simulink model "final"  (R2024b)
settings: Solver=ode23t  StartTime=0.0  StopTime=0.5  RelTol=1e-3
libraries: spsSeriesRLCBranchLib x4, spsRMSLib x2, spsCurrentMeasurementLib x1, spsDiodeLib x1, spsIGBTDiodeLib x1, spsPVArrayLib x1, slpidlib x1, simulink x1, spsVoltageMeasurementLib x1, sps_lib x1
settings Model: Creator=Aamith Kishore T J  LastModifiedBy=Aamith Kishore T J

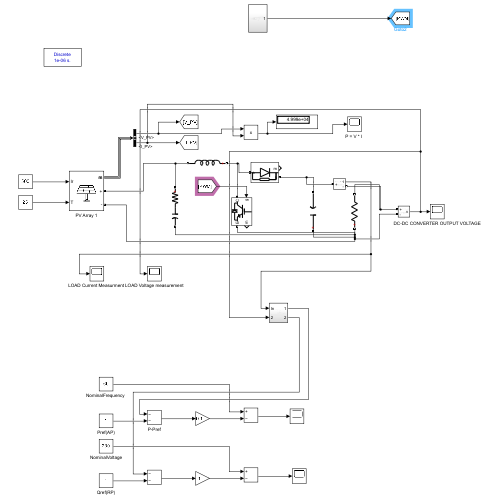
[thumbnail: Simulink's stored preview of the top-level diagram]
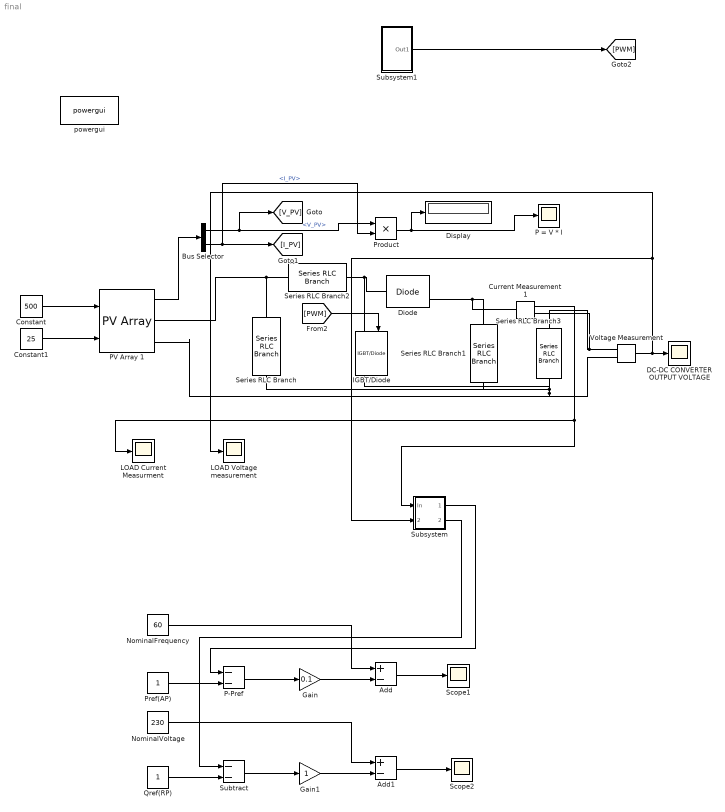
== system final ==
  Add : Sum  Inputs=+-
  Add1 : Sum  Inputs=+-
  Bus Selector : BusSelector  OutputSignals=V_PV,I_PV
  Constant : Constant  Value=500
  Constant1 : Constant  Value=25
  Current Measurement1 : spsCurrentMeasurementLib/Current Measurement  PhasorSimulation=off  OutputType=Complex  PSBequivalent=0
  DC-DC CONVERTER OUTPUT VOLTAGE : Scope
  Diode : spsDiodeLib/Diode  Ron=0.001  Lon=0  Vf=0.8  IC=0  UseSnubber=0  Rs=500  Cs=250e-9  Measurements=on
  Display : Display
  Gain : Gain  Gain=0.1
  Gain1 : Gain
  IGBT/Diode : spsIGBTDiodeLib/IGBT//Diode  Ron=1e-3  Rs=1e5  Cs=inf  Measurements=on
  "LOAD Current Measurment " : Scope
  LOAD Voltage measurement : Scope
  "NominalFrequency " : Constant  Value=60
  NominalVoltage : Constant  Value=230
  "P = V * I " : Scope
  P-Pref : Sum  Inputs=--
  PV Array 1 : spsPVArrayLib/PV Array  Npar=47  Nser=10  PlotType=array @ 25 deg.C & specified irradiances  S_vec="[ 1000  500  100 ]"  Temp_C_vec=[25 0]  ModuleName=A2Peak Power POWER ON P220-6x10  PlotWhenSelected=off  Pm=219.978  Ncell=60  Voc=36.72  Isc=7.98  Vm=30.3  Im=7.26  beta_Voc_pc=-0.35  alpha_Isc_pc=0.05  beta_Voc=-0.12852  alpha_Isc=0.00399  IL=8.0041  I0=1.8441e-10  nI=0.97472  Rsh=85.0716  Rs=0.25728  RobustModel=off  RobustCellTemperature=313.3991  BAL=on  Tc=1e-6  Tfilter=5e-5
  Pref(AP) : Constant
  Product : Product
  Qref(RP) : Constant
  Scope1 : Scope
  Scope2 : Scope
  Series RLC Branch : spsSeriesRLCBranchLib/Series RLC Branch  LConnTagsString=__new0  RConnTagsString=__new0  BranchType=RC  Resistance=0.0001  Inductance=1e-3  SetiL0=off  InitialCurrent=0  Capacitance=1000e-6  Setx0=off  InitialVoltage=0  Measurements=None
  Series RLC Branch1 : spsSeriesRLCBranchLib/Series RLC Branch  LConnTagsString=__new0  RConnTagsString=__new0  BranchType=C  Resistance=0.0001  Inductance=1.45e-6  SetiL0=off  InitialCurrent=0  Capacitance=3227e-6  Setx0=off  InitialVoltage=0  Measurements=None
  Series RLC Branch2 : spsSeriesRLCBranchLib/Series RLC Branch  LConnTagsString=__new0  RConnTagsString=__new0  BranchType=L  Resistance=0.0001  Inductance=1.45e-6  SetiL0=off  InitialCurrent=0  Capacitance=9888-6  Setx0=off  InitialVoltage=0  Measurements=None
  Series RLC Branch3 : spsSeriesRLCBranchLib/Series RLC Branch  LConnTagsString=__new0  RConnTagsString=__new0  BranchType=R  Resistance=2  Inductance=1.45e-6  SetiL0=off  InitialCurrent=0  Capacitance=3227e-6  Setx0=off  InitialVoltage=0  Measurements=None
  Subsystem : Subsystem
  Subsystem1 : Subsystem
  Subtract : Sum  Inputs=--
  Voltage Measurement : spsVoltageMeasurementLib/Voltage Measurement  PhasorSimulation=off  OutputType=Complex  PSBequivalent=0
  powergui : sps_lib/powergui  Priority=1  SimulationMode=Discrete  SampleTime=1e-6  frequency=60  Iterations=50  frequencyindice=0  Pbase=100e6  ErrMax=1e-4  UnitsV=kV  UnitsW=MW  buscounter=0  FunctionMessages=off  echomessages=off  EnableUseOfTLC=off  CurrentSourceSwitches=off  DisableSnubberDevices=off  DisableRonSwitches=off  DisableVfSwitches=off  DisplayEquations=off  AutomaticDiscreteSolvers=off  SolverType=Tustin/Backward Euler (TBE)  Interpol=off  ExternalGateDelay=off  methode=off  Ts=100  x0status=blocks  SPID=on  SwTol=0  HookPort=off  NonlinearTolerance=1e-4  nMaxIteration=100  ContinueOnMaxIteration=off  RestoreLinks=warning  ResistiveCurrentMeasurement=off  Frange=[0:2:500]  Ylog=off  Xlog=on  ShowGrid=off  save=off  variable=ZData  structure=0  ZoomFFT=off  StartTime=0.0  cycles=1  DisplayStyle=1  fundamental=60  FreqAxis=off  MaxFrequency=1000  frequencyindicesteady=1  RmsSteady=1  display=off
  wires:
  Constant/1 -> PV Array 1/1
  Constant1/1 -> PV Array 1/2
  PV Array 1/1 -> Bus Selector/1
  Bus Selector/1 -> Product/1, [V_PV]  "<V_PV>"
  Bus Selector/2 -> Product/2, [I_PV]  "<I_PV>"
  [PWM] -> IGBT/Diode/1
  Product/1 -> "P = V * I "/1, Display/1
  P-Pref/1 -> Gain/1
  Pref(AP)/1 -> P-Pref/2
  "NominalFrequency "/1 -> Add/1
  Gain/1 -> Add/2
  Add/1 -> Scope1/1
  Qref(RP)/1 -> Subtract/2
  Subtract/1 -> Gain1/1
  NominalVoltage/1 -> Add1/1
  Gain1/1 -> Add1/2
  Add1/1 -> Scope2/1
  Voltage Measurement/1 -> Subsystem/2(In1), LOAD Voltage measurement/1, DC-DC CONVERTER OUTPUT VOLTAGE/1
  Current Measurement1/1 -> Subsystem/1(In), "LOAD Current Measurment "/1
  Subsystem/1(Out1) -> P-Pref/1
  Subsystem/2(Out2) -> Subtract/1
  Subsystem1/1(Out1) -> [PWM]
  connections:
  PV Array 1/RConn1 -- Series RLC Branch2/RConn1 -- Series RLC Branch/LConn1
  Series RLC Branch/RConn1 -- Voltage Measurement/LConn2 -- PV Array 1/RConn2 -- Series RLC Branch1/LConn1 -- IGBT/Diode/RConn1 -- Series RLC Branch3/LConn1
  Diode/LConn1 -- Series RLC Branch2/LConn1 -- IGBT/Diode/LConn1
  Diode/RConn1 -- Current Measurement1/LConn1 -- Series RLC Branch1/RConn1
  Series RLC Branch3/RConn1 -- Voltage Measurement/LConn1 -- Current Measurement1/RConn1

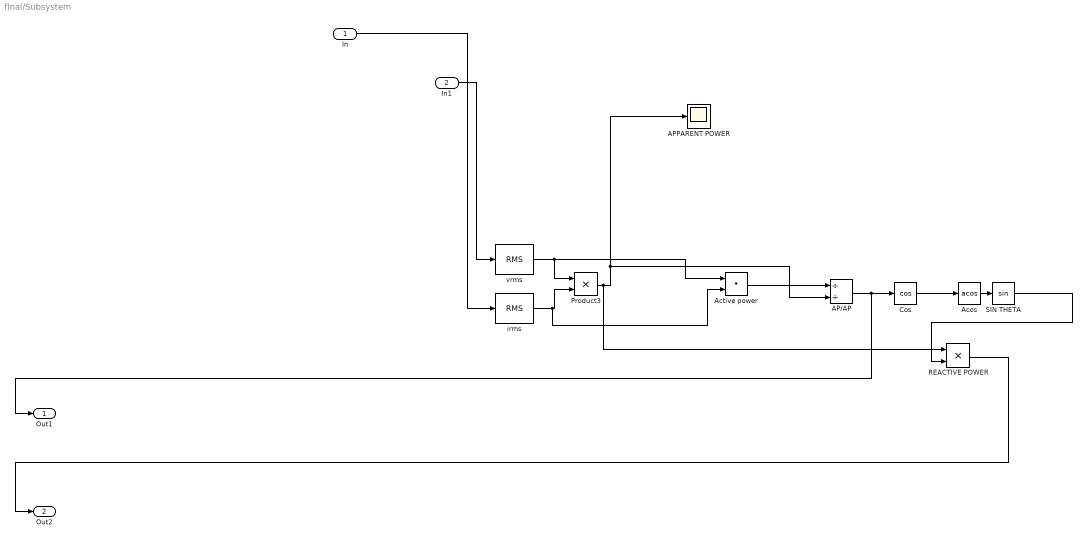
== system final/Subsystem ==
  In : Inport
  In1 : Inport  Port=2
  AP/AP : Product  Inputs=//
  APPARENT POWER : Scope
  Acos : Trigonometry  Operator=acos
  Active power : DotProduct  OutDataTypeStr=Inherit: Inherit via internal rule
  Cos : Trigonometry  Operator=cos
  Product3 : Product
  REACTIVE POWER : Product
  SIN THETA : Trigonometry
  irms : spsRMSLib/RMS  TrueRMS=on  Freq=60  RMSInit=120  Ts=0
  vrms : spsRMSLib/RMS  TrueRMS=on  Freq=60  RMSInit=120  Ts=0
  Out1 : Outport
  Out2 : Outport  Port=2
  wires:
  Acos/1 -> SIN THETA/1
  irms/1 -> Active power/2, Product3/2
  AP/AP/1 -> Out1/1, Cos/1
  vrms/1 -> Active power/1, Product3/1
  SIN THETA/1 -> REACTIVE POWER/2
  Active power/1 -> AP/AP/1
  In1/1 -> vrms/1
  Product3/1 -> REACTIVE POWER/1, AP/AP/2, APPARENT POWER/1
  REACTIVE POWER/1 -> Out2/1
  Cos/1 -> Acos/1
  In/1 -> irms/1

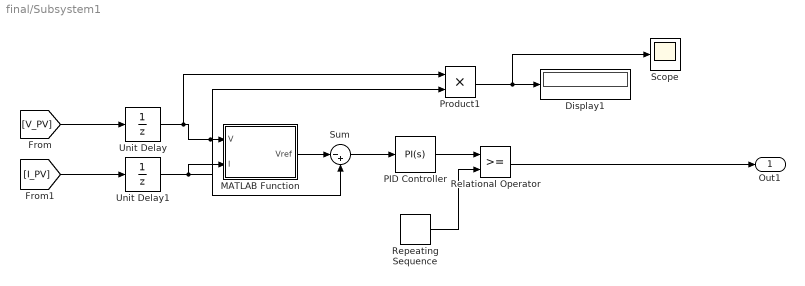
== system final/Subsystem1 ==
  Display1 : Display
  MATLAB Function : MATLAB Function  TreatAsAtomicUnit=on
  PID Controller : slpidlib/PID Controller  Controller=PI  Form=Parallel  TimeDomain=Continuous-time  UseExternalTs=off  SampleTime=-1  IntegratorMethod=Forward Euler  FilterMethod=Forward Euler  ControllerParametersSource=internal  P=0.001  I=0.01  UseKiTs=off  D=0  UseExternalDerivativeSource=off  N=100  UseFilter=on  TunerSelectOption=Transfer Function Based (PID Tuner App)  InitialConditionSource=internal  InitialConditionForIntegrator=0  InitialConditionForFilter=0  DifferentiatorICPrevScaledInput=0  ExternalReset=none  TrackingMode=off  Kt=1  LimitOutput=on  SatLimitsSource=internal  UpperSaturationLimit=0.95  LowerSaturationLimit=0  LinearizeAsGain=on  AntiWindupMode=none  Kb=1  LimitIntegrator=off  UpperIntegratorSaturationLimit=inf  LowerIntegratorSaturationLimit=-inf  POutMin=[]  POutMax=[]  IOutMin=[]  IOutMax=[]  DOutMin=[]  DOutMax=[]  NOutMin=[]  NOutMax=[]  SumOutMin=[]  SumOutMax=[]  SaturationOutMin=[]  SaturationOutMax=[]  PParamMin=[]  PParamMax=[]  IParamMin=[]  IParamMax=[]  DParamMin=[]  DParamMax=[]  NParamMin=[]  NParamMax=[]  KbParamMin=[]  KbParamMax=[]  KtParamMin=[]  KtParamMax=[]  KbOutMin=[]  KbOutMax=[]  KtOutMin=[]  KtOutMax=[]  IntegratorOutMin=[]  IntegratorOutMax=[]  FilterOutMin=[]  FilterOutMax=[]  SumI1OutMin=[]  SumI1OutMax=[]  SumI2OutMin=[]  SumI2OutMax=[]  SumI3OutMin=[]  SumI3OutMax=[]  SumI4OutMin=[]  SumI4OutMax=[]  SumDOutMin=[]  SumDOutMax=[]  DifferentiatorOutMin=[]  DifferentiatorOutMax=[]  FilterDiffOutCoefMin=[]  FilterDiffOutCoefMax=[]  ReciprocalOutMin=[]  ReciprocalOutMax=[]  SumDenOutMin=[]  SumDenOutMax=[]  SumNumOutMin=[]  SumNumOutMax=[]  DivideOutMin=[]  DivideOutMax=[]  UdiffTsProdOutMin=[]  UdiffTsProdOutMax=[]  NTsProdOutMin=[]  NTsProdOutMax=[]  UintegralTsProdOutMin=[]  UintegralTsProdOutMax=[]  UngainTsProdOutMin=[]  UngainTsProdOutMax=[]  ClampingZeroOutDataTypeStr=Inherit: Inherit via back propagation  ClampingZeroOutMin=[]  ClampingZeroOutMax=[]  FilterDenConstantOutDataTypeStr=Inherit: Inherit via back propagation  FilterDenConstantOutMin=[]  FilterDenConstantOutMax=[]  PCopyOutDataTypeStr=Inherit: Inherit via back propagation  PCopyOutMin=[]  PCopyOutMax=[]  NCopyOutDataTypeStr=Inherit: Inherit via back propagation  NCopyOutMin=[]  NCopyOutMax=[]  IntegratorContinuousStateAttributes=''  IntegratorStateMustResolveToSignalObject=off  IntegratorRTWStateStorageClass=Auto  FilterContinuousStateAttributes=''  FilterStateMustResolveToSignalObject=off  FilterRTWStateStorageClass=Auto  ParallelPVariant=InternalParameters  IdealPVariant=Disabled  IVariant=InternalParameters  DVariant=Disabled  IntegratorVariant=Continuous  SatVariant=Enabled  AWVariant=Passthrough  PCopyVariant=Disabled  TRVariant=Disabled  FdbkBlocksVariant=Forward  IdealPFdbkVariant=Disabled  SatFdbkVariant=Disabled  DerivativeFilterVariant=Disabled  NVariant=Disabled  NCopyVariant=Disabled_SignalSpec  FilterICVariant=Disabled  IntegratorICVariant=InternalICs  ExternalResetVariant=Disabled  TRSumVariant=Passthrough  SumFdbkVariant=Disabled  SumVariant=Sum_PI  TsampFilterVariant=InternalTs  TsampNgainVariant=Passthrough  TsampIntegralVariant=Disabled_SignalSpec  ExternalSaturationOutDataTypeStr=Inherit: Same as second input  DerivativeSourceVariant=Disabled  PreIntVariant=InternalPreInt
  Product1 : Product
  Relational Operator : RelationalOperator  OutDataTypeStr=boolean  RndMeth=Simplest  InputSameDT=off
  Repeating Sequence : simulink/Sources/Repeating Sequence  rep_seq_t=[0 0.0002]  rep_seq_y=[0 1]
  Scope : Scope
  Sum : Sum  Inputs=|-+
  Unit Delay : UnitDelay  SampleTime=1e-4  HasFrameUpgradeWarning=on
  Unit Delay1 : UnitDelay  SampleTime=1e-4  HasFrameUpgradeWarning=on
  Out1 : Outport
  wires:
  PID Controller/1 -> Relational Operator/1
  Unit Delay1/1 -> Product1/2, MATLAB Function/2(I)
  [I_PV] -> Unit Delay1/1
  MATLAB Function/1(Vref) -> Sum/1
  Repeating Sequence/1 -> Relational Operator/2
  Unit Delay/1 -> Product1/1, Sum/2, MATLAB Function/1(V)
  Sum/1 -> PID Controller/1
  [V_PV] -> Unit Delay/1
  Product1/1 -> Scope/1, Display1/1
  Relational Operator/1 -> Out1/1

== matlab function final/Subsystem1/MATLAB Function ==
  data: Vref output; V input; I input
function Vref = RefGen(V, I)
    % Define constants
    Vrefmax = 363;
    Vrefmin = 0;
    Vrefinit = 300;
    deltaVref = 1;
    
    % Define data type for code generation
    dataType = 'double';
    
    % Initialize persistent variables
    persistent Vold Pold Vrefold;
    if isempty(Vold)
        Vold = 0;
        Pold = 0;
        Vrefold = Vrefinit;
    end
    
    % Calculate current power
    P = V * I;
    
    % Calculate changes in voltage and power
    dV = V - Vold;
    dP = P - Pold;
    
    % Initialize Vref to the previous value as a default
    Vref = Vrefold;
    
    % Perturb and Observe logic (similar to MPPT or voltage reference adjustment)
    if dP ~= 0
        if dP < 0
            if dV < 0
                Vref = Vrefold + deltaVref; % Increase Vref if power decreases and voltage decreases
            else
                Vref = Vrefold - deltaVref; % Decrease Vref if power decreases and voltage increases
            end
        else % Handle dP > 0 (power increases)
            if dV > 0
                Vref = Vrefold + deltaVref; % Increase Vref if power and voltage increase
            else
                Vref = Vrefold - deltaVref; % Decrease Vref if power increases but voltage decreases
            end
        end
    end
    
    % Limit Vref to the specified range
    if Vref > Vrefmax
        Vref = Vrefmax;
    elseif Vref < Vrefmin
        Vref = Vrefmin;
    end
    
    % Update persistent variables
    Vrefold = Vref;
    Vold = V;
    Pold = P;
end
